simulink model "escalon"  (R2023a)
settings: Solver=VariableStepAuto  StartTime=0.0  StopTime=900  MaxStep=0.01  RelTol=1e-3
undefined symbols (not defined in the file or in its folder): ci
settings Model: Creator=pipeh  LastModifiedBy=pipeh
settings DataIOCC: SaveOutput=off  SignalLogging=off  DSMLogging=off  SaveTime=off  ReturnWorkspaceOutputs=off

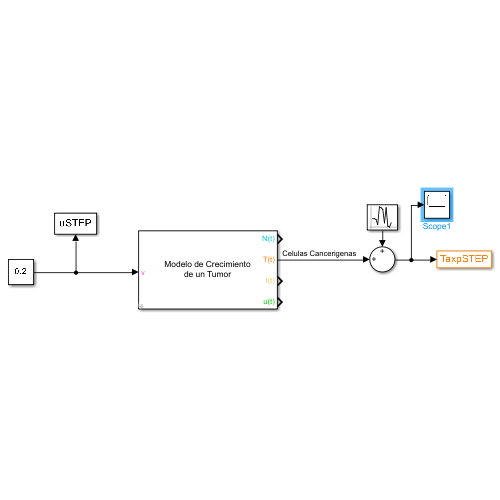
[thumbnail: Simulink's stored preview of the top-level diagram]
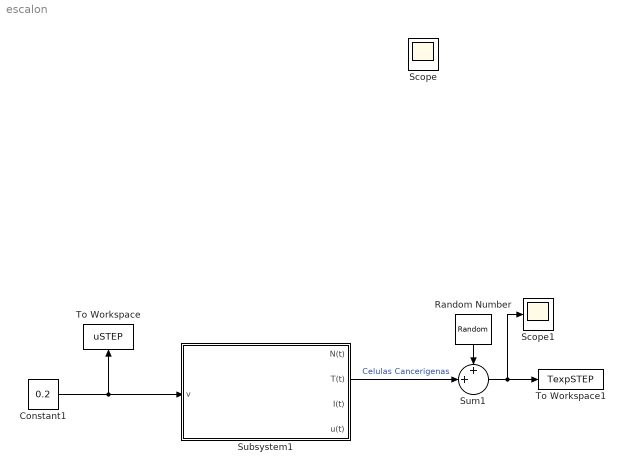
== system escalon ==
  Constant1 : Constant  Value=0.2
  Random Number : RandomNumber  Variance=0.00001  SampleTime=9
  Scope1 : Scope
  Subsystem1 : Subsystem  mask(Modelo del crecimiento de un tumor){a1=0.2, a2=0.3, a3=0.1, b1=1, b2=1, alpha=0.3, c1=1, c2=0.5, c3=1, c4=1, d1=0.2, d2=1, r1=1.5, r2=1, s=0.33, rho=0.01, N0=1, T0=0.25, I0=0.15, u0=0, ci=ci}
      mask prompts: alpha "α"; rho "ρ"; N0 "Condicion Inicial N"; T0 "Condicion Inicial T"; I0 "Condicion Inicial I"; u0 "Condicion Inicial u"; ci "Condiciones Iniciales [N(0) T(0) I(0) u(0)]"
      mask Help: parametros
      mask Display: disp("Modelo de Crecimiento\nde un Tumor")
  Sum1 : Sum  Inputs=++|
  To Workspace : ToWorkspace  VariableName=uSTEP  SampleTime=9
  To Workspace1 : ToWorkspace  VariableName=TexpSTEP  SampleTime=9
  Scope : Scope
  wires:
  Subsystem1/2(T(t)) -> Sum1/2  "Celulas Cancerigenas"
  Random Number/1 -> Sum1/1
  Sum1/1 -> Scope1/1, To Workspace1/1
  Constant1/1 -> Subsystem1/1(v), To Workspace/1

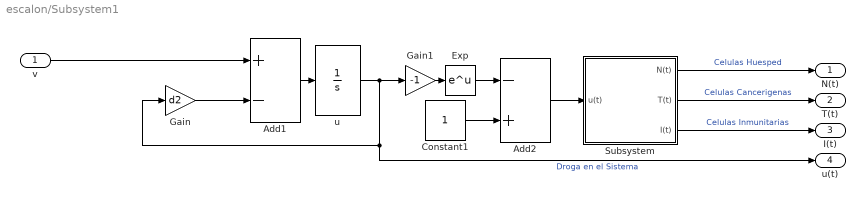
== system escalon/Subsystem1 ==
  v : Inport
  Add1 : Sum  Inputs=+-
  Add2 : Sum  Inputs=-+
  Constant1 : Constant
  Exp : Math
  Gain : Gain  Gain=d2
  Gain1 : Gain  Gain=-1
  Subsystem : Subsystem
  u : Integrator  InitialCondition=u0
  N(t) : Outport
  T(t) : Outport  Port=2
  I(t) : Outport  Port=3
  u(t) : Outport  Port=4
  wires:
  Add1/1 -> u/1
  u/1 -> Gain1/1, u(t)/1, Gain/1  "Droga en el Sistema"
  Exp/1 -> Add2/1
  Gain/1 -> Add1/2
  Add2/1 -> Subsystem/1(u(t))
  Subsystem/1(N(t)) -> N(t)/1  "Celulas Huesped"
  Constant1/1 -> Add2/2
  Subsystem/3(I(t)) -> I(t)/1  "Celulas Inmunitarias"
  Subsystem/2(T(t)) -> T(t)/1  "Celulas Cancerigenas"
  v/1 -> Add1/1
  Gain1/1 -> Exp/1

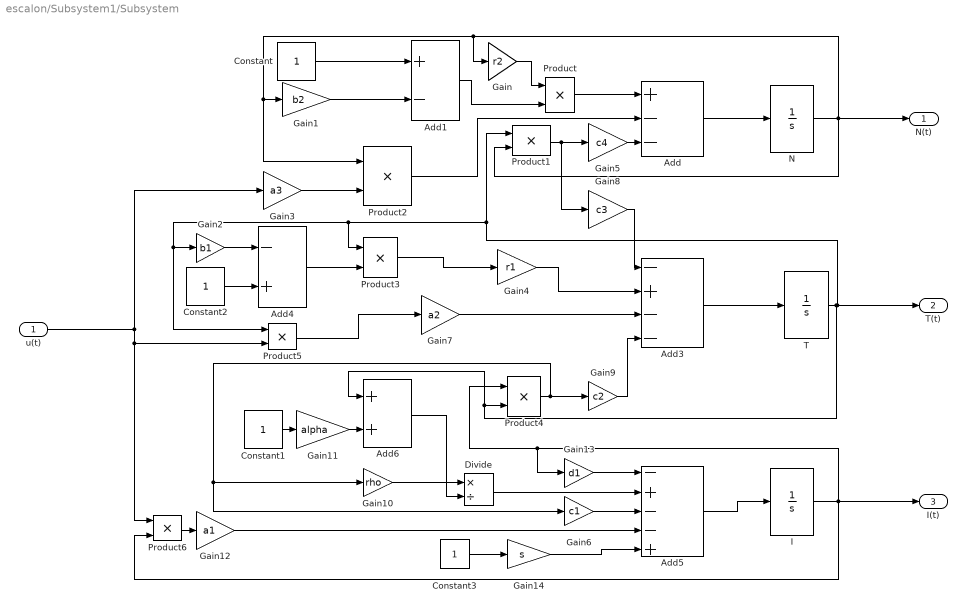
== system escalon/Subsystem1/Subsystem ==
  u(t) : Inport
  Add : Sum  Inputs=+--
  Add1 : Sum  Inputs=+-
  Add3 : Sum  Inputs=-+--
  Add4 : Sum  Inputs=-+
  Add5 : Sum  Inputs=-+--+
  Add6 : Sum
  Constant{,1..3} (4 alike) : Constant
  Divide : Product  Inputs=*/
  Gain : Gain  Gain=r2
  Gain1 : Gain  Gain=b2
  Gain10 : Gain  Gain=rho
  Gain11 : Gain  Gain=alpha
  Gain12 : Gain  Gain=a1
  Gain13 : Gain  Gain=d1
  Gain14 : Gain  Gain=s
  Gain2 : Gain  Gain=b1
  Gain3 : Gain  Gain=a3
  Gain4 : Gain  Gain=r1
  Gain5 : Gain  Gain=c4
  Gain6 : Gain  Gain=c1
  Gain7 : Gain  Gain=a2
  Gain8 : Gain  Gain=c3
  Gain9 : Gain  Gain=c2
  I : Integrator  InitialCondition=I0  LimitOutput=on  LowerSaturationLimit=0
  N : Integrator  InitialCondition=N0  LimitOutput=on  LowerSaturationLimit=0  WrappedStateLowerValue=0
  Product{,1..6} (7 alike) : Product
  T : Integrator  InitialCondition=T0  LimitOutput=on  LowerSaturationLimit=0
  N(t) : Outport
  T(t) : Outport  Port=2
  I(t) : Outport  Port=3
  wires:
  Gain12/1 -> Add5/4
  Product1/1 -> Gain8/1, Gain5/1
  Add1/1 -> Product/2
  N/1 -> Product2/1, Gain1/1, Gain/1, N(t)/1, Product1/2
  Gain/1 -> Product/1
  Gain3/1 -> Product2/2
  Product3/1 -> Gain4/1
  Gain6/1 -> Add5/3
  Add5/1 -> I/1
  Divide/1 -> Add5/2
  T/1 -> T(t)/1, Product1/1, Gain2/1, Product5/1, Product3/1, Add6/1, Product4/2
  Gain2/1 -> Add4/1
  Product2/1 -> Add/2
  I/1 -> Product6/2, I(t)/1, Gain13/1, Product4/1
  Add6/1 -> Divide/2
  Add3/1 -> T/1
  Add4/1 -> Product3/2
  Gain10/1 -> Divide/1
  Gain9/1 -> Add3/4
  Gain7/1 -> Add3/3
  Gain5/1 -> Add/3
  Product4/1 -> Gain10/1, Gain6/1, Gain9/1
  Gain1/1 -> Add1/2
  Product/1 -> Add/1
  Add/1 -> N/1
  Constant/1 -> Add1/1
  Gain4/1 -> Add3/2
  Gain8/1 -> Add3/1
  Constant2/1 -> Add4/2
  u(t)/1 -> Product6/1, Product5/2, Gain3/1
  Gain11/1 -> Add6/2
  Constant1/1 -> Gain11/1
  Gain13/1 -> Add5/1
  Constant3/1 -> Gain14/1
  Gain14/1 -> Add5/5
  Product5/1 -> Gain7/1
  Product6/1 -> Gain12/1
